simulink model "EIRSAT_ADCS"  (Simulink 8.9)
settings: Solver=VariableStepAuto  StartTime=0.0  StopTime=10.0  RelTol=1e-3
libraries: shared6dof x1
settings Model: Creator=JoeT  LastModifiedBy=JoeT
settings DataIOCC: LimitDataPoints=off  SaveFormat=Dataset  SignalLoggingSaveFormat=Dataset
settings OptimizationCC: LifeSpan=auto
settings DebuggingCC: UnderspecifiedInitializationDetection=Simplified  MergeDetectMultiDrivingBlocksExec=error  FcnCallInpInsideContextMsg=error  StateNameClashWarn=none  SFUnexpectedBacktrackingDiag=error  SFNoUnconditionalDefaultTransitionDiag=error  SFExecutionAtInitializationDiag=warning
settings HardwareCC: ProdBitPerPointer=64  ProdBitPerSizeT=64  ProdBitPerPtrDiffT=64  ProdLargestAtomicFloat=Float  ProdIntDivRoundTo=Zero  ProdEndianess=LittleEndian  ProdWordSize=64  ProdHWDeviceType=Intel->x86-64 (Windows64)
settings ModelReferenceCC: PropagateSignalLabelsOutOfModel=on
settings GRTTargetCC: TargetLangStandard=C99 (ISO)  GeneratePreprocessorConditionals=Use local settings  CombineOutputUpdateFcns=on  GRTInterface=off
settings ConfigComp: CovMetricSettings=dwe  CovHtmlReporting=off  CovSaveCumulativeToWorkspaceVar=off  CovSaveSingleToWorkspaceVar=off  CovExternalEMLEnable=on

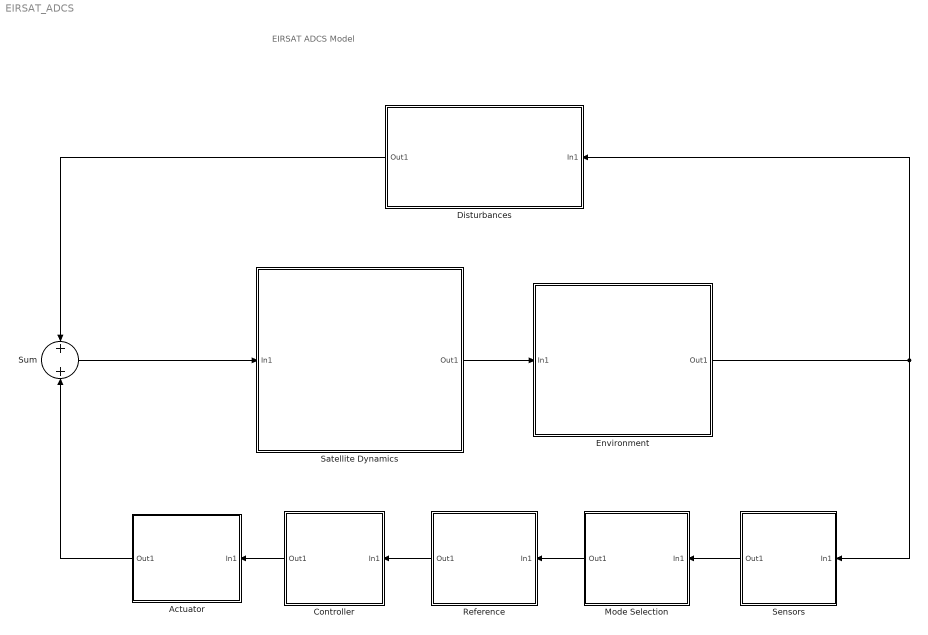
== system EIRSAT_ADCS ==
  note: EIRSAT ADCS Model
  Actuator : Subsystem  TreatAsAtomicUnit=on
  Controller : Subsystem  TreatAsAtomicUnit=on
  Disturbances : Subsystem  TreatAsAtomicUnit=on
  Environment : Subsystem  TreatAsAtomicUnit=on
  Mode Selection : Subsystem  TreatAsAtomicUnit=on
  Reference : Subsystem  TreatAsAtomicUnit=on
  Satellite Dynamics : Subsystem  TreatAsAtomicUnit=on
  Sensors : Subsystem  TreatAsAtomicUnit=on
  Sum : Sum  Inputs=+|+
  wires:
  Reference/1(Out1) -> Controller/1(In1)
  Controller/1(Out1) -> Actuator/1(In1)
  Disturbances/1(Out1) -> Sum/1
  Actuator/1(Out1) -> Sum/2
  Sum/1 -> Satellite Dynamics/1(In1)
  Mode Selection/1(Out1) -> Reference/1(In1)
  Sensors/1(Out1) -> Mode Selection/1(In1)
  Satellite Dynamics/1(Out1) -> Environment/1(In1)
  Environment/1(Out1) -> Disturbances/1(In1), Sensors/1(In1)

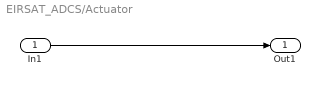
== system EIRSAT_ADCS/Actuator ==
  In1 : Inport
  Out1 : Outport
  wires:
  In1/1 -> Out1/1

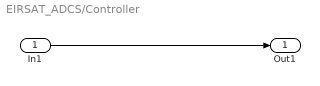
== system EIRSAT_ADCS/Controller ==
  In1 : Inport
  Out1 : Outport
  wires:
  In1/1 -> Out1/1

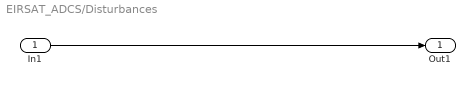
== system EIRSAT_ADCS/Disturbances ==
  In1 : Inport
  Out1 : Outport
  wires:
  In1/1 -> Out1/1

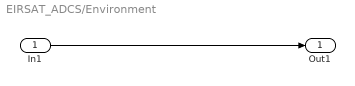
== system EIRSAT_ADCS/Environment ==
  In1 : Inport
  Out1 : Outport
  wires:
  In1/1 -> Out1/1

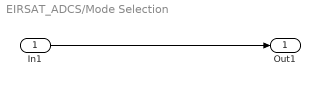
== system EIRSAT_ADCS/Mode Selection ==
  In1 : Inport
  Out1 : Outport
  wires:
  In1/1 -> Out1/1

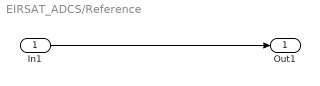
== system EIRSAT_ADCS/Reference ==
  In1 : Inport
  Out1 : Outport
  wires:
  In1/1 -> Out1/1

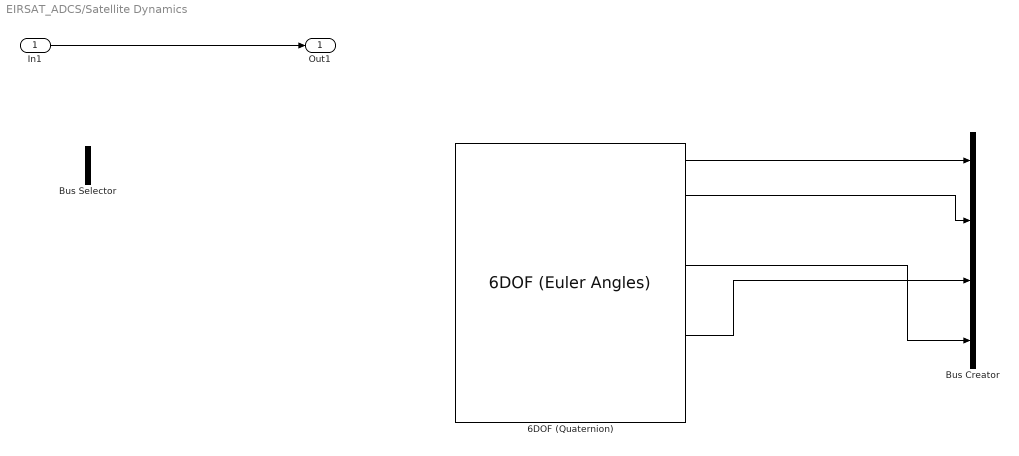
== system EIRSAT_ADCS/Satellite Dynamics ==
  In1 : Inport
  6DOF (Quaternion) : shared6dof/6DOF (Euler Angles)  units=Metric (MKS)  mtype=Fixed  rep=Quaternion  xme_0=[0 0 0]  Vm_0=[0 0 0]  eul_0=[0 0 0]  pm_0=[0 0 0]  mass_0=1.0  mass_e=0.5  mass_f=2.0  inertia=eye(3)  inertia_e=eye(3)  inertia_f=2*eye(3)  k_quat=1.0  vre_flag=on  abi_flag=off
  Bus Creator : BusCreator  Inputs=4
  Bus Selector : BusSelector  OutputSignals=signal1,signal2
  Out1 : Outport
  wires:
  In1/1 -> Out1/1
  6DOF (Quaternion)/1 -> Bus Creator/1
  6DOF (Quaternion)/2 -> Bus Creator/2
  6DOF (Quaternion)/4 -> Bus Creator/4
  6DOF (Quaternion)/6 -> Bus Creator/3

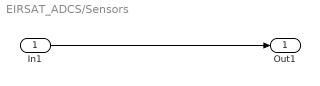
== system EIRSAT_ADCS/Sensors ==
  In1 : Inport
  Out1 : Outport
  wires:
  In1/1 -> Out1/1
